simulink model "AC_gen_SG"  (R2025a)
settings: Solver=VariableStepAuto  StartTime=0.0  StopTime=10.0  RelTol=1e-3
undefined symbols (not defined in the file): buses_lf, gen_static_params, Grid_op_SG, Matrix_flux_to_i, Ps_lf, Sb, SGs_buses, SGs_nodes
(part 2 of 2)

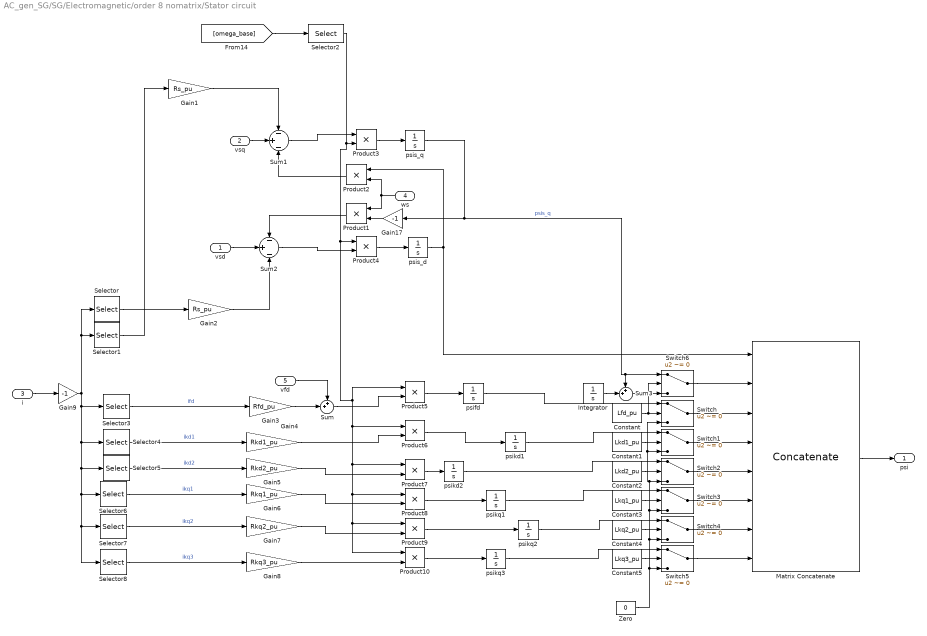
== system AC_gen_SG/SG/Electromagnetic/order 8 nomatrix/Stator circuit ==
  vsd : Inport
  vsq : Inport  Port=2
  i : Inport  Port=3
  ws : Inport  Port=4
  vfd : Inport  Port=5
  Constant : Constant  Value=Lfd_pu  VectorParams1D=off
  Constant1 : Constant  Value=Lkd1_pu  VectorParams1D=off
  Constant2 : Constant  Value=Lkd2_pu  VectorParams1D=off
  Constant3 : Constant  Value=Lkq1_pu  VectorParams1D=off
  Constant4 : Constant  Value=Lkq2_pu  VectorParams1D=off
  Constant5 : Constant  Value=Lkq3_pu  VectorParams1D=off
  Gain1 : Gain  Gain=Rs_pu
  Gain17 : Gain  Gain=-1
  Gain2 : Gain  Gain=Rs_pu
  Gain3 : Gain  Gain=Rfd_pu
  Gain4 : Gain  Gain=Rkd1_pu
  Gain5 : Gain  Gain=Rkd2_pu
  Gain6 : Gain  Gain=Rkq1_pu
  Gain7 : Gain  Gain=Rkq2_pu
  Gain8 : Gain  Gain=Rkq3_pu
  Gain9 : Gain  Gain=-1
  Integrator : Integrator  InitialCondition=Grid_op_SG.op.States(6).x'
  Matrix Concatenate : Concatenate  NumInputs=8  Mode=Multidimensional array
  Product{1..10} (10 alike) : Product
  Selector : Selector  NumberOfDimensions=2  InputPortWidth=9  IndexOptions=Index vector (dialog),Select all  Indices=[1],1  OutputSizes=1,1
  Selector1 : Selector  NumberOfDimensions=2  InputPortWidth=9  IndexOptions=Index vector (dialog),Select all  Indices=[2],1  OutputSizes=1,1
  Selector2 : Selector  InputPortWidth=length(fref.ref_units)  IndexOptions=Index vector (dialog)  Indices=block_fref  OutputSizes=1
  Selector3 : Selector  NumberOfDimensions=2  InputPortWidth=9  IndexOptions=Index vector (dialog),Select all  Indices=3,1  OutputSizes=1,1
  Selector4 : Selector  NumberOfDimensions=2  InputPortWidth=9  IndexOptions=Index vector (dialog),Select all  Indices=4,1  OutputSizes=1,1
  Selector5 : Selector  NumberOfDimensions=2  InputPortWidth=9  IndexOptions=Index vector (dialog),Select all  Indices=5,1  OutputSizes=1,1
  Selector6 : Selector  NumberOfDimensions=2  InputPortWidth=9  IndexOptions=Index vector (dialog),Select all  Indices=6,1  OutputSizes=1,1
  Selector7 : Selector  NumberOfDimensions=2  InputPortWidth=9  IndexOptions=Index vector (dialog),Select all  Indices=7,1  OutputSizes=1,1
  Selector8 : Selector  NumberOfDimensions=2  InputPortWidth=9  IndexOptions=Index vector (dialog),Select all  Indices=8,1  OutputSizes=1,1
  Sum : Sum  Inputs=++|
  Sum1 : Sum  Inputs=-|+|-  InputSameDT=on  SaturateOnIntegerOverflow=on  OutDataTypeStr=Inherit: Same as first input
  Sum2 : Sum  Inputs=-|+|-  InputSameDT=on  SaturateOnIntegerOverflow=on  OutDataTypeStr=Inherit: Same as first input
  Sum3 : Sum  Inputs=++|
  Switch{,1..6} (7 alike) : Switch  Criteria=u2 ~= 0  SaturateOnIntegerOverflow=off  InputSameDT=off
  Zero : Constant  Value=0  OutDataTypeStr=Inherit: Inherit via back propagation
  psifd : Integrator  InitialCondition=Grid_op_SG.op.States(7).x'
  psikd1 : Integrator  InitialCondition=Grid_op_SG.op.States(8).x'
  psikd2 : Integrator  InitialCondition=Grid_op_SG.op.States(9).x'
  psikq1 : Integrator  InitialCondition=Grid_op_SG.op.States(10).x'
  psikq2 : Integrator  InitialCondition=Grid_op_SG.op.States(11).x'
  psikq3 : Integrator  InitialCondition=Grid_op_SG.op.States(12).x'
  psis_d : Integrator  InitialCondition=Grid_op_SG.op.States(13).x'
  psis_q : Integrator  InitialCondition=Grid_op_SG.op.States(14).x'
  psi : Outport  VectorParamsAs1DForOutWhenUnconnected=off
  wires:
  Sum3/1 -> Switch6/3
  Integrator/1 -> Sum3/2
  Switch6/1 -> Matrix Concatenate/2
  Constant5/1 -> Switch5/2
  Constant4/1 -> Switch4/2
  Constant3/1 -> Switch3/2
  Constant2/1 -> Switch2/2
  Constant1/1 -> Switch1/2
  psikq3/1 -> Switch5/1
  psikq2/1 -> Switch4/1
  psikq1/1 -> Switch3/1
  psikd2/1 -> Switch2/1
  psikd1/1 -> Switch1/1
  Switch4/1 -> Matrix Concatenate/7
  Switch5/1 -> Matrix Concatenate/8
  Switch3/1 -> Matrix Concatenate/6
  Switch2/1 -> Matrix Concatenate/5
  Switch1/1 -> Matrix Concatenate/4
  Zero/1 -> Switch5/3, Switch4/3, Switch3/3, Switch2/3, Switch1/3, Switch/3
  psifd/1 -> Switch/1
  Constant/1 -> Switch/2, Switch6/2
  Product5/1 -> psifd/1
  Switch/1 -> Matrix Concatenate/3
  Gain5/1 -> Product7/2
  Selector2/1 -> Product3/2, Product4/1, Product5/1, Product6/1, Product7/1, Product8/1, Product9/1, Product10/1
  [omega_base] -> Selector2/1
  vsq/1 -> Sum1/2
  Gain1/1 -> Sum1/1
  Selector1/1 -> Gain1/1
  Gain2/1 -> Sum2/3
  Selector/1 -> Gain2/1
  psis_d/1 -> Matrix Concatenate/1, Product2/1
  Product2/1 -> Sum1/3
  Product1/1 -> Sum2/1
  psis_q/1 -> Gain17/1, Switch6/1, Sum3/1  "psis_q"
  Gain17/1 -> Product1/2
  ws/1 -> Product2/2, Product1/1
  Product4/1 -> psis_d/1
  Sum2/1 -> Product4/2
  vsd/1 -> Sum2/2
  Gain9/1 -> Selector/1, Selector1/1, Selector3/1, Selector4/1, Selector5/1, Selector6/1, Selector7/1, Selector8/1
  Product10/1 -> psikq3/1
  Product9/1 -> psikq2/1
  Product8/1 -> psikq1/1
  Product7/1 -> psikd2/1
  Product6/1 -> psikd1/1
  i/1 -> Gain9/1
  Matrix Concatenate/1 -> psi/1
  Gain7/1 -> Product9/2
  Gain8/1 -> Product10/2
  Gain6/1 -> Product8/2
  Gain4/1 -> Product6/2
  Sum/1 -> Product5/2
  vfd/1 -> Sum/1
  Gain3/1 -> Sum/2
  Selector4/1 -> Gain4/1  "ikd1"
  Selector5/1 -> Gain5/1  "ikd2"
  Selector6/1 -> Gain6/1  "ikq1"
  Selector7/1 -> Gain7/1  "ikq2"
  Selector8/1 -> Gain8/1  "ikq3"
  Selector3/1 -> Gain3/1  "ifd"
  Sum1/1 -> Product3/1
  Product3/1 -> psis_q/1

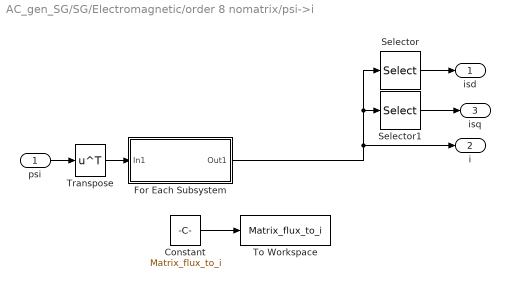
== system AC_gen_SG/SG/Electromagnetic/order 8 nomatrix/psi->i ==
  psi : Inport
  Constant : Constant  Value=Matrix_flux_to_i
  For Each Subsystem : Subsystem  TreatAsAtomicUnit=on  mask{Matrix_flux_to_i=Matrix_flux_to_i}
  Selector : Selector  NumberOfDimensions=2  InputPortWidth=9  IndexOptions=Index vector (dialog),Select all  Indices=[1],1  OutputSizes=1,1
  Selector1 : Selector  NumberOfDimensions=2  InputPortWidth=9  IndexOptions=Index vector (dialog),Select all  Indices=[2],1  OutputSizes=1,1
  To Workspace : ToWorkspace  VariableName=Matrix_flux_to_i  SaveFormat=Timeseries  SampleTime=-1
  Transpose : Math  Operator=transpose
  isd : Outport  VectorParamsAs1DForOutWhenUnconnected=off
  i : Outport  Port=2  VectorParamsAs1DForOutWhenUnconnected=off
  isq : Outport  Port=3  VectorParamsAs1DForOutWhenUnconnected=off
  wires:
  Constant/1 -> To Workspace/1
  For Each Subsystem/1(Out1) -> i/1, Selector/1, Selector1/1
  Transpose/1 -> For Each Subsystem/1(In1)
  Selector1/1 -> isq/1
  psi/1 -> Transpose/1
  Selector/1 -> isd/1

== system AC_gen_SG/SG/Electromagnetic/order 8 nomatrix/psi->i/For Each Subsystem ==
  In1 : Inport  Partition=on  PartitionDimension=1  PartitionWidth=1  PartitionOffset=0
  For Each : ForEach  DisableCoverage=on  IterateSubsysMaskParameter=on  SubsysMaskParameterIterationDimension=3
  Gain : Gain  Gain=Matrix_flux_to_i  Multiplication=Matrix(K*u)
  Out1 : Outport  ConcatenationDimension=2
  wires:
  Gain/1 -> Out1/1
  In1/1 -> Gain/1
